simulink library "sm_wheel_loader_lib"  (R2026a)
settings: Solver=VariableStepAuto
undefined symbols (not defined in the file): AToTOrificeVector, BiPOrificeVector, boomHEArea, boomREArea, BToTOrificeVector, fluids, GRake, GToothL, GToothR, HMPST, HydFcnParams, logLoad, Position, PToAOrificeVector, PToBOrificeVector, RakeL, RakeR, testInput, Wheel_Loader, X, Y, Z
libraries: sm_lib x694, fl_lib x183, nesl_utility x74, SimscapeFluids_lib x62, sdl_lib x25, cvt_components_lib x25, simulink_extras x5, $bdroot x4, wheel_loader_contact_lib x4, ee_lib x2, SignalEditorBlockLib x1, batteryecm_lib x1
(part 5 of 25)

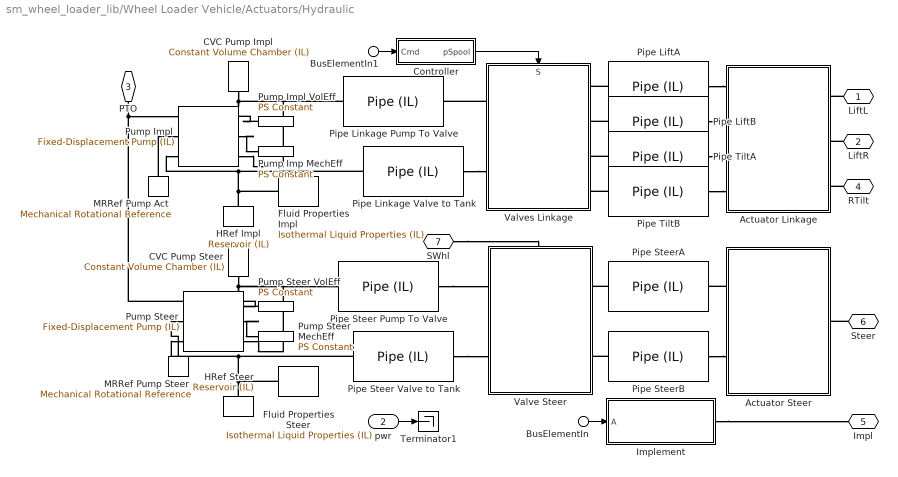
== system sm_wheel_loader_lib/Wheel Loader Vehicle/Actuators/Hydraulic ==
  BusElementIn : Inport  PortName=Cmd  Element=Actuator
  BusElementIn1 : Inport  PortName=Cmd  Element=Operator
  pwr : Inport  Port=2
  Actuator Linkage : Subsystem
      mask Display: image('sm_wheel_loader_actuator_linkage_IMAGE.png');
  Actuator Steer : Subsystem
      mask Display: image('sm_wheel_loader_actuator_steer_IMAGE.png');
  CVC Pump Impl : fl_lib/Isothermal Liquid/Elements/Constant Volume Chamber (IL)  volume=HydFcnParams.pump.chamberVol mm^3  p_I_specify=off  p_I_priority=High  p_I=0.101325 MPa  p_I_nominal_specify=off  p_I_nominal_value=1  p_I_nominal_unit=MPa
  CVC Pump Steer : fl_lib/Isothermal Liquid/Elements/Constant Volume Chamber (IL)  volume=HydFcnParams.steerPump.chamberVol mm^3  p_I_specify=off  p_I_priority=High  p_I=0.101325 MPa  p_I_nominal_specify=off  p_I_nominal_value=1  p_I_nominal_unit=MPa
  Controller : Subsystem
  Fluid Properties Impl : fl_lib/Isothermal Liquid/Utilities/Isothermal Liquid Properties (IL)  rho_L_atm=870 kg/m^3  bulk_modulus_model=foundation.enum.bulk_modulus_model.const  beta_gain=6  beta_L_atm=1.45e9 Pa  nu_atm=46 mm^2/s  p_atm=0.101325 MPa  p_min=0.1 Pa  properties_range_check=simscape.enum.assert.action.error  air_fraction=0.005  polytropic_index=1.0  rho_g_atm=1.225 kg/m^3  air_dissolution_model=simscape.enum.onoff.off  p_crit=3 MPa
  Fluid Properties Steer : fl_lib/Isothermal Liquid/Utilities/Isothermal Liquid Properties (IL)  rho_L_atm=870 kg/m^3  bulk_modulus_model=foundation.enum.bulk_modulus_model.const  beta_gain=6  beta_L_atm=1.45e9 Pa  nu_atm=46 mm^2/s  p_atm=0.101325 MPa  p_min=0.1 Pa  properties_range_check=simscape.enum.assert.action.error  air_fraction=0.005  polytropic_index=1.0  rho_g_atm=1.225 kg/m^3  air_dissolution_model=simscape.enum.onoff.off  p_crit=3 MPa
  HRef Impl : fl_lib/Isothermal Liquid/Elements/Reservoir (IL)  pressure_input=false  pressure_spec=foundation.enum.pressure_spec.atmospheric  reservoir_pressure=0.101325 MPa
  HRef Steer : fl_lib/Isothermal Liquid/Elements/Reservoir (IL)  pressure_input=false  pressure_spec=foundation.enum.pressure_spec.atmospheric  reservoir_pressure=0.101325 MPa
  Implement : Subsystem  Variant=on  VariantControlMode=label  VariantControl=Grapple Rake  LabelModeActiveChoice=Bucket
      settings: AttributesFormatString=%<LabelModeActiveChoice>
  MRRef Pump Act : fl_lib/Mechanical/Rotational Elements/Mechanical Rotational Reference
  MRRef Pump Steer : fl_lib/Mechanical/Rotational Elements/Mechanical Rotational Reference
  Pipe LiftA : fl_lib/Isothermal Liquid/Elements/Pipe (IL)  length=HydFcnParams.pipes.length mm  area=HydFcnParams.pipe.crossSectArea mm^2  Dh=HydFcnParams.pipes.hydraulicDiam mm  length_add=1 m  roughness=15e-6 m  Re_lam=2000  Re_tur=4000  shape_factor=64  dynamic_compressibility=simscape.enum.onoff.off  inertia=simscape.enum.onoff.off  p0=0.101325 MPa  mdot0=0 kg/s
  Pipe LiftB : fl_lib/Isothermal Liquid/Elements/Pipe (IL)  length=HydFcnParams.pipes.length mm  area=HydFcnParams.pipe.crossSectArea mm^2  Dh=HydFcnParams.pipes.hydraulicDiam mm  length_add=1 m  roughness=15e-6 m  Re_lam=2000  Re_tur=4000  shape_factor=64  dynamic_compressibility=simscape.enum.onoff.off  inertia=simscape.enum.onoff.off  p0=0.101325 MPa  mdot0=0 kg/s
  Pipe Linkage Pump To Valve : fl_lib/Isothermal Liquid/Elements/Pipe (IL)  length=HydFcnParams.pipes.length mm  area=HydFcnParams.pipe.crossSectArea mm^2  Dh=HydFcnParams.pipes.hydraulicDiam mm  length_add=1 m  roughness=15e-6 m  Re_lam=2000  Re_tur=4000  shape_factor=64  dynamic_compressibility=simscape.enum.onoff.off  inertia=simscape.enum.onoff.off  p0=0.101325 MPa  mdot0=0 kg/s
  Pipe Linkage Valve to Tank : fl_lib/Isothermal Liquid/Elements/Pipe (IL)  length=HydFcnParams.pipes.length mm  area=HydFcnParams.pipe.crossSectArea mm^2  Dh=HydFcnParams.pipes.hydraulicDiam mm  length_add=1 m  roughness=15e-6 m  Re_lam=2000  Re_tur=4000  shape_factor=64  dynamic_compressibility=simscape.enum.onoff.off  inertia=simscape.enum.onoff.off  p0=0.101325 MPa  mdot0=0 kg/s
  Pipe Steer Pump To Valve : fl_lib/Isothermal Liquid/Elements/Pipe (IL)  length=HydFcnParams.pipes.length mm  area=HydFcnParams.pipe.crossSectArea mm^2  Dh=HydFcnParams.pipes.hydraulicDiam mm  length_add=1 m  roughness=15e-6 m  Re_lam=2000  Re_tur=4000  shape_factor=64  dynamic_compressibility=simscape.enum.onoff.off  inertia=simscape.enum.onoff.off  p0=0.101325 MPa  mdot0=0 kg/s
  Pipe Steer Valve to Tank : fl_lib/Isothermal Liquid/Elements/Pipe (IL)  length=HydFcnParams.pipes.length mm  area=HydFcnParams.pipe.crossSectArea mm^2  Dh=HydFcnParams.pipes.hydraulicDiam mm  length_add=1 m  roughness=15e-6 m  Re_lam=2000  Re_tur=4000  shape_factor=64  dynamic_compressibility=simscape.enum.onoff.off  inertia=simscape.enum.onoff.off  p0=0.101325 MPa  mdot0=0 kg/s
  Pipe SteerA : fl_lib/Isothermal Liquid/Elements/Pipe (IL)  length=HydFcnParams.pipes.length mm  area=HydFcnParams.pipe.crossSectArea mm^2  Dh=HydFcnParams.pipes.hydraulicDiam mm  length_add=1 m  roughness=15e-6 m  Re_lam=2000  Re_tur=4000  shape_factor=64  dynamic_compressibility=simscape.enum.onoff.off  inertia=simscape.enum.onoff.off  p0=0.101325 MPa  mdot0=0 kg/s
  Pipe SteerB : fl_lib/Isothermal Liquid/Elements/Pipe (IL)  length=HydFcnParams.pipes.length mm  area=HydFcnParams.pipe.crossSectArea mm^2  Dh=HydFcnParams.pipes.hydraulicDiam mm  length_add=1 m  roughness=15e-6 m  Re_lam=2000  Re_tur=4000  shape_factor=64  dynamic_compressibility=simscape.enum.onoff.off  inertia=simscape.enum.onoff.off  p0=0.101325 MPa  mdot0=0 kg/s
  Pipe TiltA : fl_lib/Isothermal Liquid/Elements/Pipe (IL)  length=HydFcnParams.pipes.length mm  area=HydFcnParams.pipe.crossSectArea mm^2  Dh=HydFcnParams.pipes.hydraulicDiam mm  length_add=1 m  roughness=15e-6 m  Re_lam=2000  Re_tur=4000  shape_factor=64  dynamic_compressibility=simscape.enum.onoff.off  inertia=simscape.enum.onoff.off  p0=0.101325 MPa  mdot0=0 kg/s
  Pipe TiltB : fl_lib/Isothermal Liquid/Elements/Pipe (IL)  length=HydFcnParams.pipes.length mm  area=HydFcnParams.pipe.crossSectArea mm^2  Dh=HydFcnParams.pipes.hydraulicDiam mm  length_add=1 m  roughness=15e-6 m  Re_lam=2000  Re_tur=4000  shape_factor=64  dynamic_compressibility=simscape.enum.onoff.off  inertia=simscape.enum.onoff.off  p0=0.101325 MPa  mdot0=0 kg/s
  Pump Impl : SimscapeFluids_lib/Isothermal Liquid/Pumps & Motors/Fixed-Displacement Pump (IL)  leakage_friction_spec=fluids.isothermal_liquid.pumps_motors.enum.pump_motor_loss_spec.input_efficiency  displacement=HydFcnParams.pump.displacement cm^3/rev  omega_nominal=HydFcnParams.pump.nomSpeed rpm  p_nominal=HydFcnParams.pump.nomPrGain bar  vol_eff_nominal=HydFcnParams.pump.volEff  mech_eff_nominal=HydFcnParams.pump.mechEff  no_load_torque=0 N*m  p_diff_eff_TLU=[.1, 1, 2] MPa  omega_eff_TLU=[250, 500, 1000, 2000, 3000, 4000] rpm  vol_eff_TLU=[.816, .908, .954, .977, .981, .984; .325, .663, .831, .916, .925, .946; .137, .568, .78, .892, .893, .91]  mech_eff_TLU=[.996, .996, .996, .996, .996, .996; .988, .989, .989, .989, .989, .99; .981, .981, .982, .982, .983, .984]  p_diff_loss_TLU=[.1, 1, 2] MPa  omega_loss_TLU=[250, 500, 1000, 2000, 3000, 4000] rpm  vol_loss_TLU=1e-3 * [.023, .023, .023, .023, .0285, .032; .0844, .0842, .0845, .084, .1125, .108; .1079, .108, .11, .108, .1605, .18] m^3/s  mech_loss_TLU=[.002, .002, .002, .002, .002, .002; .0607, .0556, .0556, .0556, .0556, .0505; .1937, .1937, .1833, .1833, .1729, .1626] N*m  vol_eff_min=1e-3  vol_eff_max=1  mech_eff_min=1e-3  mech_eff_max=1  pressure_threshold=1e-3 MPa  omega_threshold=100 rpm  supplied_range_check=simscape.enum.assert.action.none  pump_mode_check=simscape.enum.assert.action.none  pressure_check=simscape.enum.assert.action.none  p_min_valid=0.101325 MPa
  Pump Steer : SimscapeFluids_lib/Isothermal Liquid/Pumps & Motors/Fixed-Displacement Pump (IL)  leakage_friction_spec=fluids.isothermal_liquid.pumps_motors.enum.pump_motor_loss_spec.input_efficiency  displacement=HydFcnParams.steerPump.displacement cm^3/rev  omega_nominal=HydFcnParams.pump.nomSpeed rpm  p_nominal=HydFcnParams.pump.nomPrGain bar  vol_eff_nominal=HydFcnParams.pump.volEff  mech_eff_nominal=HydFcnParams.pump.mechEff  no_load_torque=0 N*m  p_diff_eff_TLU=[.1, 1, 2] MPa  omega_eff_TLU=[250, 500, 1000, 2000, 3000, 4000] rpm  vol_eff_TLU=[.816, .908, .954, .977, .981, .984; .325, .663, .831, .916, .925, .946; .137, .568, .78, .892, .893, .91]  mech_eff_TLU=[.996, .996, .996, .996, .996, .996; .988, .989, .989, .989, .989, .99; .981, .981, .982, .982, .983, .984]  p_diff_loss_TLU=[.1, 1, 2] MPa  omega_loss_TLU=[250, 500, 1000, 2000, 3000, 4000] rpm  vol_loss_TLU=1e-3 * [.023, .023, .023, .023, .0285, .032; .0844, .0842, .0845, .084, .1125, .108; .1079, .108, .11, .108, .1605, .18] m^3/s  mech_loss_TLU=[.002, .002, .002, .002, .002, .002; .0607, .0556, .0556, .0556, .0556, .0505; .1937, .1937, .1833, .1833, .1729, .1626] N*m  vol_eff_min=1e-3  vol_eff_max=1  mech_eff_min=1e-3  mech_eff_max=1  pressure_threshold=1e-3 MPa  omega_threshold=100 rpm  supplied_range_check=simscape.enum.assert.action.none  pump_mode_check=simscape.enum.assert.action.none  pressure_check=simscape.enum.assert.action.none  p_min_valid=0.101325 MPa
  Pump Imp MechEff : fl_lib/Physical Signals/Sources/PS Constant  constant=HydFcnParams.pump.mechEff
  Pump Impl VolEff : fl_lib/Physical Signals/Sources/PS Constant  constant=HydFcnParams.pump.volEff
  Pump Steer MechEff : fl_lib/Physical Signals/Sources/PS Constant  constant=HydFcnParams.steerPump.mechEff
  Pump Steer VolEff : fl_lib/Physical Signals/Sources/PS Constant  constant=HydFcnParams.steerPump.volEff
  Terminator1 : Terminator
  Valve Steer : Subsystem
      settings: PortSchema="{\"entries\":[{\"content\":{\"sides\":[{\"content\":{\"connectorIds\":[\"LConn1\",\"LConn2\"]},\"type\":\"ConnectorPlacement.EquallySpacedRectSide\",\"uuid\":\"408e1035-6b3d-4519-b3f1-e009707ee901\"},{\"content\":{\"connectorIds\":[\"RConn1\",\"RConn2\"],\"side\":\"RIGHT\"},\"type\":\"ConnectorPlacement.EquallySpacedRectSide\",\"uuid\":\"f6fc5ec3-963d-4896-a810-4c1d83a284ca\"},{\"content\":{\"connectorIds\":[\"LConn3\"],\"side\":\"TOP\"},\"type\":\"ConnectorPlacement.EquallySpacedRectSide\",\"uuid\":\"5ee59ebc-e402-4785-9120-6ae47dd60b43\"},{\"content\":{\"side\":\"BOTTOM\"},\"type\":\"ConnectorPlacement.EquallySpacedRectSide\",\"uuid\":\"a994d606-c935-4c5d-b566-9fce03890d2a\"}]},\"type\":\"ConnectorPlacement.EquallySpacedConnector\",\"uuid\":\"c6791463-b308-429c-8dd1-d15f50199213\"}],\"packageUris\":[\"http://schema.mathworks.com/mf0/Connector/R2020b\"],\"version\":\"1.0\"}"
      mask Display: image('sm_wheel_loader_valve_gerotor_IMAGE.png');
  Valves Linkage : Subsystem
      settings: PortSchema="{\"entries\":[{\"content\":{\"sides\":[{\"content\":{\"connectorIds\":[\"LConn1\",\"LConn2\"]},\"type\":\"ConnectorPlacement.EquallySpacedRectSide\",\"uuid\":\"e97bc73b-9f55-4fad-8581-2066e0d00398\"},{\"content\":{\"connectorIds\":[\"RConn1\",\"RConn2\",\"RConn3\",\"RConn4\"],\"side\":\"RIGHT\"},\"type\":\"ConnectorPlacement.EquallySpacedRectSide\",\"uuid\":\"96a7ce6b-69e5-4ab0-8b6a-18f7c232fee9\"},{\"content\":{\"connectorIds\":[\"In1\"],\"side\":\"TOP\"},\"type\":\"ConnectorPlacement.EquallySpacedRectSide\",\"uuid\":\"ae84efc8-1053-4ca4-8a9f-7b6269b642b7\"}]},\"type\":\"ConnectorPlacement.EquallySpacedConnector\",\"uuid\":\"dc6a267f-cf26-460c-b9d1-1342509ba07b\"}],\"packageUris\":[\"http://schema.mathworks.com/mf0/Connector/R2020b\"],\"version\":\"1.0\"}"
      mask Display: image('sm_wheel_loader_valve_linkage_IMAGE.png');
  LiftL : PMIOPort  Side=Right
  LiftR : PMIOPort  Port=2  Side=Right
  PTO : PMIOPort  Port=3  Side=Left
  RTilt : PMIOPort  Port=4  Side=Left
  Impl : PMIOPort  Port=5  Side=Right
  Steer : PMIOPort  Port=6  Side=Right
  SWhl : PMIOPort  Port=7  Side=Left
  wires:
  BusElementIn1/1 -> Controller/1(Cmd)
  BusElementIn/1 -> Implement/1(A)
  Controller/1(pSpool) -> Valves Linkage/1(S)
  pwr/1 -> Terminator1/1
  connections:
  Pump Steer/RConn1 -- Pump Impl/RConn1 -- PTO/RConn1
  Implement/RConn1 -- Impl/RConn1
  Steer/RConn1 -- Actuator Steer/RConn1
  LiftR/RConn1 -- Actuator Linkage/RConn2
  MRRef Pump Steer/LConn1 -- Pump Steer/RConn2
  MRRef Pump Act/LConn1 -- Pump Impl/RConn2
  Pipe Steer Pump To Valve/RConn1 -- Valve Steer/LConn1
  Pump Steer/LConn2 -- Pump Steer MechEff/RConn1
  Pump Steer VolEff/RConn1 -- Pump Steer/LConn1
  Pipe Steer Valve to Tank/LConn1 -- Valve Steer/LConn2
  CVC Pump Steer/LConn1 -- Pump Steer/LConn3 -- Pipe Steer Pump To Valve/LConn1
  Fluid Properties Steer/RConn1 -- Pipe Steer Valve to Tank/RConn1 -- Pump Steer/RConn3 -- HRef Steer/LConn1
  Pipe SteerB/LConn1 -- Valve Steer/RConn2
  Pipe SteerA/LConn1 -- Valve Steer/RConn1
  RTilt/RConn1 -- Actuator Linkage/RConn3
  Actuator Steer/LConn1 -- Pipe SteerA/RConn1
  Pipe SteerB/RConn1 -- Actuator Steer/LConn2
  Pipe TiltB/RConn1 -- Actuator Linkage/LConn4
  Pipe TiltA/RConn1 -- Actuator Linkage/LConn3
  Pipe LiftB/RConn1 -- Actuator Linkage/LConn2
  Pipe LiftA/RConn1 -- Actuator Linkage/LConn1
  LiftL/RConn1 -- Actuator Linkage/RConn1
  Pipe TiltB/LConn1 -- Valves Linkage/RConn4
  Pipe TiltA/LConn1 -- Valves Linkage/RConn3
  Pipe LiftB/LConn1 -- Valves Linkage/RConn2
  Pipe LiftA/LConn1 -- Valves Linkage/RConn1
  Pipe Linkage Valve to Tank/LConn1 -- Valves Linkage/LConn2
  Valves Linkage/LConn1 -- Pipe Linkage Pump To Valve/RConn1
  HRef Impl/LConn1 -- Pipe Linkage Valve to Tank/RConn1 -- Pump Impl/RConn3 -- Fluid Properties Impl/RConn1
  Pipe Linkage Pump To Valve/LConn1 -- Pump Impl/LConn3 -- CVC Pump Impl/LConn1
  Pump Impl/LConn2 -- Pump Imp MechEff/RConn1
  Pump Impl VolEff/RConn1 -- Pump Impl/LConn1
  SWhl/RConn1 -- Valve Steer/LConn3

== system sm_wheel_loader_lib/Wheel Loader Vehicle/Actuators/Ideal ==
  note: The actuation of the cylinders is done through prescribed motion at the joints.
  Cmd : Inport
  pwr : Inport  Port=2
  Power Draw : Subsystem
  Shaft Inertia : fl_lib/Mechanical/Rotational Elements/Inertia  inertia=0.01 kg*m^2  num_ports=foundation.enum.numPorts2.one  w_specify=on  w_priority=None  w=0 rad/s  w_nominal_specify=off  w_nominal_value=1  w_nominal_unit=rad/s  t_specify=off  t_priority=None  t=0 N*m  t_nominal_specify=off  t_nominal_value=1  t_nominal_unit=N*m
  Steering Mechanism Inertia : fl_lib/Mechanical/Rotational Elements/Inertia  inertia=0.01 kg*m^2  num_ports=foundation.enum.numPorts2.one  w_specify=off  w_priority=High  w=0 rad/s  w_nominal_specify=off  w_nominal_value=1  w_nominal_unit=rad/s  t_specify=off  t_priority=None  t=0 N*m  t_nominal_specify=off  t_nominal_value=1  t_nominal_unit=N*m
  Terminator : Terminator
  LiftL : PMIOPort  Side=Right
  LiftR : PMIOPort  Port=2  Side=Right
  PTO : PMIOPort  Port=3  Side=Left
  RTilt : PMIOPort  Port=4  Side=Left
  Impl : PMIOPort  Port=5  Side=Right
  Steer : PMIOPort  Port=6  Side=Right
  SWhl : PMIOPort  Port=7  Side=Left
  wires:
  Cmd/1 -> Terminator/1
  pwr/1 -> Power Draw/1(pwr)
  connections:
  PTO/RConn1 -- Power Draw/RConn1 -- Shaft Inertia/LConn1
  Steering Mechanism Inertia/LConn1 -- SWhl/RConn1

== system sm_wheel_loader_lib/Wheel Loader Vehicle/Driveline/Axle Housing Front ==
  Bearing : sm_lib/Body Elements/File Solid  ExtGeomFileName=AxleF_Housing_Bearing.STEP  UnitType=FromFile  ExtGeomFileUnits=m  StepReaderType=HEX  ExportConvexHullGeometry=off  InertiaType=Custom  BasedOnType=DensityFromFile  Density=1000  DensityUnits=kg/m^3  Mass=Wheel_Loader.bodyGroups(36).subGroups(2).inertialProperties.mass  MassUnits=kg  CenterOfMass=Wheel_Loader.bodyGroups(36).subGroups(2).inertialProperties.centerOfMass  CenterOfMassUnits=m  MomentsOfInertia=Wheel_Loader.bodyGroups(36).subGroups(2).inertialProperties.momentsOfInertia  MomentsOfInertiaUnits=kg*m^2  ProductsOfInertia=Wheel_Loader.bodyGroups(36).subGroups(2).inertialProperties.productsOfInertia  ProductsOfInertiaUnits=kg*m^2  GraphicType=FromGeometry  MarkerShape=Sphere  MarkerSize=10  GraphicVisPropType=SimpleVisualProperties  GraphicDiffuseColor=Wheel_Loader.bodyGroups(36).subGroups(2).visualProperties.rgb  GraphicOpacity=fa_casing_opc  GraphicSpecularColor=[0.5 0.5 0.5 1.0]  GraphicAmbientColor=[0.15 0.15 0.15 1.0]  GraphicEmissiveColor=[0.0 0.0 0.0 1.0]  GraphicShininess=75  DoExposeReferenceFrame=on  SerializedFrames=<Frames/>
  Bolts : sm_lib/Body Elements/File Solid  ExtGeomFileName=AxleF_Housing_Bolts.STEP  UnitType=FromFile  ExtGeomFileUnits=m  StepReaderType=HEX  ExportConvexHullGeometry=off  InertiaType=Custom  BasedOnType=DensityFromFile  Density=1000  DensityUnits=kg/m^3  Mass=Wheel_Loader.bodyGroups(36).subGroups(3).inertialProperties.mass  MassUnits=kg  CenterOfMass=Wheel_Loader.bodyGroups(36).subGroups(3).inertialProperties.centerOfMass  CenterOfMassUnits=m  MomentsOfInertia=Wheel_Loader.bodyGroups(36).subGroups(3).inertialProperties.momentsOfInertia  MomentsOfInertiaUnits=kg*m^2  ProductsOfInertia=Wheel_Loader.bodyGroups(36).subGroups(3).inertialProperties.productsOfInertia  ProductsOfInertiaUnits=kg*m^2  GraphicType=FromGeometry  MarkerShape=Sphere  MarkerSize=10  GraphicVisPropType=SimpleVisualProperties  GraphicDiffuseColor=Wheel_Loader.bodyGroups(36).subGroups(3).visualProperties.rgb  GraphicOpacity=fa_casing_opc  GraphicSpecularColor=[0.5 0.5 0.5 1.0]  GraphicAmbientColor=[0.15 0.15 0.15 1.0]  GraphicEmissiveColor=[0.0 0.0 0.0 1.0]  GraphicShininess=75  DoExposeReferenceFrame=on  SerializedFrames=<Frames/>
  Housing : sm_lib/Body Elements/File Solid  ExtGeomFileName=AxleF_Housing.STEP  UnitType=FromFile  ExtGeomFileUnits=m  StepReaderType=HEX  ExportConvexHullGeometry=off  InertiaType=Custom  BasedOnType=DensityFromFile  Density=1000  DensityUnits=kg/m^3  Mass=Wheel_Loader.bodyGroups(36).subGroups(1).inertialProperties.mass  MassUnits=kg  CenterOfMass=Wheel_Loader.bodyGroups(36).subGroups(1).inertialProperties.centerOfMass  CenterOfMassUnits=m  MomentsOfInertia=Wheel_Loader.bodyGroups(36).subGroups(1).inertialProperties.momentsOfInertia  MomentsOfInertiaUnits=kg*m^2  ProductsOfInertia=Wheel_Loader.bodyGroups(36).subGroups(1).inertialProperties.productsOfInertia  ProductsOfInertiaUnits=kg*m^2  GraphicType=FromGeometry  MarkerShape=Sphere  MarkerSize=10  GraphicVisPropType=SimpleVisualProperties  GraphicDiffuseColor=Wheel_Loader.bodyGroups(36).subGroups(1).visualProperties.rgb  GraphicOpacity=fa_casing_opc  GraphicSpecularColor=[0.5 0.5 0.5 1.0]  GraphicAmbientColor=[0.15 0.15 0.15 1.0]  GraphicEmissiveColor=[0.0 0.0 0.0 1.0]  GraphicShininess=75  DoExposeReferenceFrame=on  SerializedFrames=<Frames/>
  RT_FrontAxle_FDPinion : sm_lib/Frames and Transforms/Rigid Transform  RotationMethod=RotationMatrix  FollAlignAxisA=+X  BaseAlignAxisA=+Y  FollAlignAxisB=+Y  BaseAlignAxisB=+Z  RotationStandardAxis=+Z  RotationAngle=0.0  RotationAngleUnits=deg  RotationArbitraryAxis=[0 0 1]  RotationSequenceAxes=FollowerAxes  RotationSequence=XYX  RotationSequenceAngles=[0 0 0]  RotationSequenceAnglesUnits=deg  RotationMatrix=Wheel_Loader.coordSys(44).transform.rotation  Quaternion=[1 0 0 0]  TranslationMethod=Cartesian  TranslationCartesianOffset=Wheel_Loader.coordSys(44).transform.translation  TranslationCartesianOffsetUnits=m  TranslationStandardAxis=+Z  TranslationStandardOffset=0  TranslationStandardOffsetUnits=m  TranslationROffset=0  TranslationROffsetUnits=m  TranslationThetaOffset=0  TranslationThetaOffsetUnits=deg  TranslationZOffset=0  TranslationZOffsetUnits=m
  RT_FrontAxle_LFFDRing_Weld : sm_lib/Frames and Transforms/Rigid Transform  RotationMethod=RotationMatrix  FollAlignAxisA=+X  BaseAlignAxisA=+Y  FollAlignAxisB=+Y  BaseAlignAxisB=+Z  RotationStandardAxis=+Z  RotationAngle=0.0  RotationAngleUnits=deg  RotationArbitraryAxis=[0 0 1]  RotationSequenceAxes=FollowerAxes  RotationSequence=XYX  RotationSequenceAngles=[0 0 0]  RotationSequenceAnglesUnits=deg  RotationMatrix=Wheel_Loader.coordSys(70).transform.rotation  Quaternion=[1 0 0 0]  TranslationMethod=Cartesian  TranslationCartesianOffset=Wheel_Loader.coordSys(70).transform.translation  TranslationCartesianOffsetUnits=m  TranslationStandardAxis=+Z  TranslationStandardOffset=0  TranslationStandardOffsetUnits=m  TranslationROffset=0  TranslationROffsetUnits=m  TranslationThetaOffset=0  TranslationThetaOffsetUnits=deg  TranslationZOffset=0  TranslationZOffsetUnits=m
  RT_FrontAxle_RFFDRing_Weld : sm_lib/Frames and Transforms/Rigid Transform  RotationMethod=RotationMatrix  FollAlignAxisA=+X  BaseAlignAxisA=+Y  FollAlignAxisB=+Y  BaseAlignAxisB=+Z  RotationStandardAxis=+Z  RotationAngle=0.0  RotationAngleUnits=deg  RotationArbitraryAxis=[0 0 1]  RotationSequenceAxes=FollowerAxes  RotationSequence=XYX  RotationSequenceAngles=[0 0 0]  RotationSequenceAnglesUnits=deg  RotationMatrix=Wheel_Loader.coordSys(66).transform.rotation  Quaternion=[1 0 0 0]  TranslationMethod=Cartesian  TranslationCartesianOffset=Wheel_Loader.coordSys(66).transform.translation  TranslationCartesianOffsetUnits=m  TranslationStandardAxis=+Z  TranslationStandardOffset=0  TranslationStandardOffsetUnits=m  TranslationROffset=0  TranslationROffsetUnits=m  TranslationThetaOffset=0  TranslationThetaOffsetUnits=deg  TranslationZOffset=0  TranslationZOffsetUnits=m
  RT_FrontFrame_Axle_Weld : sm_lib/Frames and Transforms/Rigid Transform  RotationMethod=RotationMatrix  FollAlignAxisA=+X  BaseAlignAxisA=+Y  FollAlignAxisB=+Y  BaseAlignAxisB=+Z  RotationStandardAxis=+Z  RotationAngle=0.0  RotationAngleUnits=deg  RotationArbitraryAxis=[0 0 1]  RotationSequenceAxes=FollowerAxes  RotationSequence=XYX  RotationSequenceAngles=[0 0 0]  RotationSequenceAnglesUnits=deg  RotationMatrix=[1 0 0; 0 1 0; 0 0 1]  Quaternion=[1 0 0 0]  TranslationMethod=Cartesian  TranslationCartesianOffset=[0 0 0]  TranslationCartesianOffsetUnits=m  TranslationStandardAxis=+Z  TranslationStandardOffset=0  TranslationStandardOffsetUnits=m  TranslationROffset=0  TranslationROffsetUnits=m  TranslationThetaOffset=0  TranslationThetaOffsetUnits=deg  TranslationZOffset=0  TranslationZOffsetUnits=m
  HFL : PMIOPort  Side=Left
  Frame : PMIOPort  Port=2  Side=Right
  HFP : PMIOPort  Port=3  Side=Left
  HFR : PMIOPort  Port=4  Side=Left
  connections:
  RT_FrontAxle_LFFDRing_Weld/RConn1 -- HFL/RConn1
  RT_FrontAxle_RFFDRing_Weld/RConn1 -- HFR/RConn1
  RT_FrontAxle_FDPinion/RConn1 -- HFP/RConn1
  RT_FrontFrame_Axle_Weld/RConn1 -- Frame/RConn1
  Housing/RConn1 -- Bolts/RConn1 -- Bearing/RConn1 -- RT_FrontFrame_Axle_Weld/LConn1 -- RT_FrontAxle_FDPinion/LConn1 -- RT_FrontAxle_RFFDRing_Weld/LConn1 -- RT_FrontAxle_LFFDRing_Weld/LConn1

== system sm_wheel_loader_lib/Wheel Loader Vehicle/Driveline/Axle Housing Rear ==
  Bolts : sm_lib/Body Elements/File Solid  ExtGeomFileName=AxleR_Housing_Bolts.STEP  UnitType=FromFile  ExtGeomFileUnits=m  StepReaderType=HEX  ExportConvexHullGeometry=off  InertiaType=Custom  BasedOnType=DensityFromFile  Density=1000  DensityUnits=kg/m^3  Mass=Wheel_Loader.bodyGroups(37).subGroups(2).inertialProperties.mass  MassUnits=kg  CenterOfMass=Wheel_Loader.bodyGroups(37).subGroups(2).inertialProperties.centerOfMass  CenterOfMassUnits=m  MomentsOfInertia=Wheel_Loader.bodyGroups(37).subGroups(2).inertialProperties.momentsOfInertia  MomentsOfInertiaUnits=kg*m^2  ProductsOfInertia=Wheel_Loader.bodyGroups(37).subGroups(2).inertialProperties.productsOfInertia  ProductsOfInertiaUnits=kg*m^2  GraphicType=FromGeometry  MarkerShape=Sphere  MarkerSize=10  GraphicVisPropType=SimpleVisualProperties  GraphicDiffuseColor=Wheel_Loader.bodyGroups(37).subGroups(2).visualProperties.rgb  GraphicOpacity=ra_casing_opc  GraphicSpecularColor=[0.5 0.5 0.5 1.0]  GraphicAmbientColor=[0.15 0.15 0.15 1.0]  GraphicEmissiveColor=[0.0 0.0 0.0 1.0]  GraphicShininess=75  DoExposeReferenceFrame=on  SerializedFrames=<Frames/>
  Housing : sm_lib/Body Elements/File Solid  ExtGeomFileName=AxleR_Housing.STEP  UnitType=FromFile  ExtGeomFileUnits=m  StepReaderType=HEX  ExportConvexHullGeometry=off  InertiaType=Custom  BasedOnType=DensityFromFile  Density=1000  DensityUnits=kg/m^3  Mass=Wheel_Loader.bodyGroups(37).subGroups(1).inertialProperties.mass  MassUnits=kg  CenterOfMass=Wheel_Loader.bodyGroups(37).subGroups(1).inertialProperties.centerOfMass  CenterOfMassUnits=m  MomentsOfInertia=Wheel_Loader.bodyGroups(37).subGroups(1).inertialProperties.momentsOfInertia  MomentsOfInertiaUnits=kg*m^2  ProductsOfInertia=Wheel_Loader.bodyGroups(37).subGroups(1).inertialProperties.productsOfInertia  ProductsOfInertiaUnits=kg*m^2  GraphicType=FromGeometry  MarkerShape=Sphere  MarkerSize=10  GraphicVisPropType=SimpleVisualProperties  GraphicDiffuseColor=Wheel_Loader.bodyGroups(37).subGroups(1).visualProperties.rgb  GraphicOpacity=ra_casing_opc  GraphicSpecularColor=[0.5 0.5 0.5 1.0]  GraphicAmbientColor=[0.15 0.15 0.15 1.0]  GraphicEmissiveColor=[0.0 0.0 0.0 1.0]  GraphicShininess=75  DoExposeReferenceFrame=on  SerializedFrames=<Frames/>
  RT_RearAxle_GBHousing_Weld : sm_lib/Frames and Transforms/Rigid Transform  RotationMethod=RotationMatrix  FollAlignAxisA=+X  BaseAlignAxisA=+Y  FollAlignAxisB=+Y  BaseAlignAxisB=+Z  RotationStandardAxis=+Z  RotationAngle=0.0  RotationAngleUnits=deg  RotationArbitraryAxis=[0 0 1]  RotationSequenceAxes=FollowerAxes  RotationSequence=XYX  RotationSequenceAngles=[0 0 0]  RotationSequenceAnglesUnits=deg  RotationMatrix=Wheel_Loader.coordSys(56).transform.rotation  Quaternion=[1 0 0 0]  TranslationMethod=Cartesian  TranslationCartesianOffset=Wheel_Loader.coordSys(56).transform.translation  TranslationCartesianOffsetUnits=m  TranslationStandardAxis=+Z  TranslationStandardOffset=0  TranslationStandardOffsetUnits=m  TranslationROffset=0  TranslationROffsetUnits=m  TranslationThetaOffset=0  TranslationThetaOffsetUnits=deg  TranslationZOffset=0  TranslationZOffsetUnits=m
  RT_RearAxle_LRFDRing_Weld : sm_lib/Frames and Transforms/Rigid Transform  RotationMethod=RotationMatrix  FollAlignAxisA=+X  BaseAlignAxisA=+Y  FollAlignAxisB=+Y  BaseAlignAxisB=+Z  RotationStandardAxis=+Z  RotationAngle=0.0  RotationAngleUnits=deg  RotationArbitraryAxis=[0 0 1]  RotationSequenceAxes=FollowerAxes  RotationSequence=XYX  RotationSequenceAngles=[0 0 0]  RotationSequenceAnglesUnits=deg  RotationMatrix=Wheel_Loader.coordSys(62).transform.rotation  Quaternion=[1 0 0 0]  TranslationMethod=Cartesian  TranslationCartesianOffset=Wheel_Loader.coordSys(62).transform.translation  TranslationCartesianOffsetUnits=m  TranslationStandardAxis=+Z  TranslationStandardOffset=0  TranslationStandardOffsetUnits=m  TranslationROffset=0  TranslationROffsetUnits=m  TranslationThetaOffset=0  TranslationThetaOffsetUnits=deg  TranslationZOffset=0  TranslationZOffsetUnits=m
  RT_RearAxle_RRFDRing_Weld : sm_lib/Frames and Transforms/Rigid Transform  RotationMethod=RotationMatrix  FollAlignAxisA=+X  BaseAlignAxisA=+Y  FollAlignAxisB=+Y  BaseAlignAxisB=+Z  RotationStandardAxis=+Z  RotationAngle=0.0  RotationAngleUnits=deg  RotationArbitraryAxis=[0 0 1]  RotationSequenceAxes=FollowerAxes  RotationSequence=XYX  RotationSequenceAngles=[0 0 0]  RotationSequenceAnglesUnits=deg  RotationMatrix=Wheel_Loader.coordSys(58).transform.rotation  Quaternion=[1 0 0 0]  TranslationMethod=Cartesian  TranslationCartesianOffset=Wheel_Loader.coordSys(58).transform.translation  TranslationCartesianOffsetUnits=m  TranslationStandardAxis=+Z  TranslationStandardOffset=0  TranslationStandardOffsetUnits=m  TranslationROffset=0  TranslationROffsetUnits=m  TranslationThetaOffset=0  TranslationThetaOffsetUnits=deg  TranslationZOffset=0  TranslationZOffsetUnits=m
  RT_RearFrame_Axle_Weld : sm_lib/Frames and Transforms/Rigid Transform  RotationMethod=RotationMatrix  FollAlignAxisA=+X  BaseAlignAxisA=+Y  FollAlignAxisB=+Y  BaseAlignAxisB=+Z  RotationStandardAxis=+Z  RotationAngle=0.0  RotationAngleUnits=deg  RotationArbitraryAxis=[0 0 1]  RotationSequenceAxes=FollowerAxes  RotationSequence=XYX  RotationSequenceAngles=[0 0 0]  RotationSequenceAnglesUnits=deg  RotationMatrix=[1 0 0; 0 1 0; 0 0 1]  Quaternion=[1 0 0 0]  TranslationMethod=Cartesian  TranslationCartesianOffset=[0 0 0]  TranslationCartesianOffsetUnits=m  TranslationStandardAxis=+Z  TranslationStandardOffset=0  TranslationStandardOffsetUnits=m  TranslationROffset=0  TranslationROffsetUnits=m  TranslationThetaOffset=0  TranslationThetaOffsetUnits=deg  TranslationZOffset=0  TranslationZOffsetUnits=m
  Frame : PMIOPort  Side=Left
  HRL : PMIOPort  Port=2  Side=Right
  HRP : PMIOPort  Port=3  Side=Right
  HRR : PMIOPort  Port=4  Side=Right
  connections:
  RT_RearAxle_LRFDRing_Weld/RConn1 -- HRL/RConn1
  RT_RearAxle_RRFDRing_Weld/RConn1 -- HRR/RConn1
  RT_RearAxle_GBHousing_Weld/RConn1 -- HRP/RConn1
  RT_RearFrame_Axle_Weld/RConn1 -- Frame/RConn1
  RT_RearAxle_RRFDRing_Weld/LConn1 -- RT_RearAxle_LRFDRing_Weld/LConn1 -- Housing/RConn1 -- Bolts/RConn1 -- RT_RearFrame_Axle_Weld/LConn1 -- RT_RearAxle_GBHousing_Weld/LConn1

== system sm_wheel_loader_lib/Wheel Loader Vehicle/Driveline/Driveline ==
  Driveline 1D : Subsystem  VariantControl=Driveline_1D
      settings: PortSchema="{\"entries\":[{\"content\":{\"sides\":[{\"content\":{\"connectorIds\":[\"LConn1\",\"LConn2\",\"LConn3\"]},\"type\":\"ConnectorPlacement.EquallySpacedRectSide\",\"uuid\":\"b63b559c-62bd-445e-b7ec-d91a1cc2405e\"},{\"content\":{\"connectorIds\":[\"RConn1\",\"RConn2\",\"RConn3\"],\"side\":\"RIGHT\"},\"type\":\"ConnectorPlacement.EquallySpacedRectSide\",\"uuid\":\"032d5054-ea2a-4303-8f34-205eab6388de\"},{\"content\":{\"connectorIds\":[\"LConn4\",\"LConn5\",\"LConn6\"],\"side\":\"TOP\"},\"type\":\"ConnectorPlacement.EquallySpacedRectSide\",\"uuid\":\"d2f0756e-9d37-498a-a5f3-0e74497a6223\"},{\"content\":{\"connectorIds\":[\"RConn4\",\"RConn5\",\"RConn6\"],\"side\":\"BOTTOM\"},\"type\":\"ConnectorPlacement.EquallySpacedRectSide\",\"uuid\":\"6a60c5c4-76fc-4699-b9fc-b8ae6c8913a6\"}]},\"type\":\"ConnectorPlacement.EquallySpacedConnector\",\"uuid\":\"1dc94a05-d7e7-41ec-b5c7-4a84600f46a8\"}],\"packageUris\":[\"http://schema.mathworks.com/mf0/Connector/R2020b\"],\"version\":\"1.0\"}"
      mask Display: image('sm_wheel_loader_driveline1D_IMAGE.png')
  Driveline 3D : Subsystem  VariantControl=Driveline_3D  mask{popup_driveJointF=CV Joint, popup_driveJointR=CV Joint}
      mask prompts: popup_driveJointF "Driveshaft Joint (front)"; popup_driveJointR "Driveshaft Joint (rear)"
      settings: PortSchema="{\"entries\":[{\"content\":{\"sides\":[{\"content\":{\"connectorIds\":[\"LConn1\",\"LConn2\",\"LConn3\"]},\"type\":\"ConnectorPlacement.EquallySpacedRectSide\",\"uuid\":\"ac94f403-7500-4d3b-9e0f-075c8f20a849\"},{\"content\":{\"connectorIds\":[\"RConn1\",\"RConn2\",\"RConn3\"],\"side\":\"RIGHT\"},\"type\":\"ConnectorPlacement.EquallySpacedRectSide\",\"uuid\":\"0eb844aa-00af-4edc-a570-50ab4e6b66c2\"},{\"content\":{\"connectorIds\":[\"LConn4\",\"LConn5\",\"LConn6\"],\"side\":\"TOP\"},\"type\":\"ConnectorPlacement.EquallySpacedRectSide\",\"uuid\":\"abddfcb0-9899-4667-9404-ac15e4716921\"},{\"content\":{\"connectorIds\":[\"RConn4\",\"RConn5\",\"RConn6\"],\"side\":\"BOTTOM\"},\"type\":\"ConnectorPlacement.EquallySpacedRectSide\",\"uuid\":\"a33fa760-6818-409d-ace3-b40bc7e3acff\"}]},\"type\":\"ConnectorPlacement.EquallySpacedConnector\",\"uuid\":\"2bc03850-1261-46ce-b9b6-2dbda85e9fb0\"}],\"packageUris\":[\"http://schema.mathworks.com/mf0/Connector/R2020b\"],\"version\":\"1.0\"}"
      mask TypeOptions popup_driveJointF:
      | Driveshaft
      | Front/popup_driveJointF
      mask TypeOptions popup_driveJointR:
      | Driveshaft
      | Rear/popup_driveJointR
      mask Display: image('sm_wheel_loader_driveline3D_IMAGE.png')
  wRL : PMIOPort  Side=Left
  Tr1 : PMIOPort  Port=2  Side=Left
  wFL : PMIOPort  Port=3  Side=Left
  HRL : PMIOPort  Port=4  Side=Left
  HRP : PMIOPort  Port=5  Side=Left
  HRR : PMIOPort  Port=6  Side=Left
  wRR : PMIOPort  Port=7  Side=Right
  Tr : PMIOPort  Port=8  Side=Right
  wFR : PMIOPort  Port=9  Side=Right
  HFL : PMIOPort  Port=10  Side=Right
  HFP : PMIOPort  Port=11  Side=Right
  HFR : PMIOPort  Port=12  Side=Right

== system sm_wheel_loader_lib/Wheel Loader Vehicle/Driveline/Wheel FL ==
  Hub : Subsystem  Tag=B230D770-3EF4-C446-A53F-6306E8DE466B
  Tire : Subsystem  Tag=1B5B75A7-7B5C-4849-8411-0061864F750D
  C : PMIOPort  Side=Left
  S : PMIOPort  Port=2  Side=Right
  connections:
  S/RConn1 -- Hub/LConn1
  Tire/LConn1 -- Hub/RConn1
  C/RConn1 -- Tire/RConn1

== system sm_wheel_loader_lib/Wheel Loader Vehicle/Driveline/Wheel FR ==
  Hub : Subsystem  Tag=5DF5B1C3-69E9-F644-9747-64BA6A51FD34
  Tire : Subsystem  Tag=2A7E39F9-3B28-3A4E-B0C7-8D7EA453C230
  S : PMIOPort  Side=Left
  C : PMIOPort  Port=2  Side=Right
  connections:
  S/RConn1 -- Hub/LConn1
  C/RConn1 -- Tire/RConn1
  Tire/LConn1 -- Hub/RConn1

== system sm_wheel_loader_lib/Wheel Loader Vehicle/Driveline/Wheel RL ==
  Hub : Subsystem  Tag=CC0284A2-2BFF-0E47-890D-925832CDD082
  Tire : Subsystem  Tag=72D24446-88E9-5644-B0BB-80BAAAD3866B
  C : PMIOPort  Side=Left
  S : PMIOPort  Port=2  Side=Right
  connections:
  C/RConn1 -- Tire/RConn1
  Tire/LConn1 -- Hub/RConn1
  S/RConn1 -- Hub/LConn1

== system sm_wheel_loader_lib/Wheel Loader Vehicle/Driveline/Wheel RR ==
  Hub : Subsystem  Tag=11A7BD13-C7ED-8E4B-96CC-E8FBD77457E9
  Tire : Subsystem  Tag=1C442381-0767-DA43-BB70-3697AC20F422
  S : PMIOPort  Side=Left
  C : PMIOPort  Port=2  Side=Right
  connections:
  S/RConn1 -- Hub/LConn1
  C/RConn1 -- Tire/RConn1
  Hub/RConn1 -- Tire/LConn1

== system sm_wheel_loader_lib/Wheel Loader Vehicle/Frame Front/Camera Frames ==
  Reference Camera Cab : sm_lib/Frames and Transforms/Reference Frame
  Reference Camera ImplRR : sm_lib/Frames and Transforms/Reference Frame
  Reference Camera IsoFR : sm_lib/Frames and Transforms/Reference Frame
  Reference Camera LinkageR : sm_lib/Frames and Transforms/Reference Frame
  Reference Camera RR : sm_lib/Frames and Transforms/Reference Frame
  Reference Camera Rear : sm_lib/Frames and Transforms/Reference Frame
  Reference Camera Right : sm_lib/Frames and Transforms/Reference Frame
  Reference Camera Roof : sm_lib/Frames and Transforms/Reference Frame
  Reference Camera WhlFR : sm_lib/Frames and Transforms/Reference Frame
  Transform Camera Cab : sm_lib/Frames and Transforms/Rigid Transform  RotationMethod=None  FollAlignAxisA=+X  BaseAlignAxisA=+Y  FollAlignAxisB=+Y  BaseAlignAxisB=+Z  RotationStandardAxis=+Z  RotationAngle=0.0  RotationAngleUnits=deg  RotationArbitraryAxis=[0 0 1]  RotationSequenceAxes=FollowerAxes  RotationSequence=XYX  RotationSequenceAngles=[0 0 0]  RotationSequenceAnglesUnits=deg  RotationMatrix=[1 0 0; 0 1 0; 0 0 1]  Quaternion=[1 0 0 0]  TranslationMethod=Cartesian  TranslationCartesianOffset=[0 -0.75 1]  TranslationCartesianOffsetUnits=m  TranslationStandardAxis=+Z  TranslationStandardOffset=0  TranslationStandardOffsetUnits=m  TranslationROffset=0  TranslationROffsetUnits=m  TranslationThetaOffset=0  TranslationThetaOffsetUnits=deg  TranslationZOffset=0  TranslationZOffsetUnits=m
  Transform Camera ImplRR : sm_lib/Frames and Transforms/Rigid Transform  RotationMethod=StandardAxis  FollAlignAxisA=+X  BaseAlignAxisA=+Y  FollAlignAxisB=+Y  BaseAlignAxisB=+Z  RotationStandardAxis=+Z  RotationAngle=+15+90  RotationAngleUnits=deg  RotationArbitraryAxis=[0 0 1]  RotationSequenceAxes=FollowerAxes  RotationSequence=XYX  RotationSequenceAngles=[0 0 0]  RotationSequenceAnglesUnits=deg  RotationMatrix=[1 0 0; 0 1 0; 0 0 1]  Quaternion=[1 0 0 0]  TranslationMethod=Cartesian  TranslationCartesianOffset=[1.0 -0.5 0.75]  TranslationCartesianOffsetUnits=m  TranslationStandardAxis=+Z  TranslationStandardOffset=0  TranslationStandardOffsetUnits=m  TranslationROffset=0  TranslationROffsetUnits=m  TranslationThetaOffset=0  TranslationThetaOffsetUnits=deg  TranslationZOffset=0  TranslationZOffsetUnits=m
  Transform Camera IsoFR : sm_lib/Frames and Transforms/Rigid Transform  RotationMethod=RotationSequence  FollAlignAxisA=+X  BaseAlignAxisA=+Y  FollAlignAxisB=+Y  BaseAlignAxisB=+Z  RotationStandardAxis=+Z  RotationAngle=0.0  RotationAngleUnits=deg  RotationArbitraryAxis=[0 0 1]  RotationSequenceAxes=FollowerAxes  RotationSequence=ZYX  RotationSequenceAngles=[45 -20 0]  RotationSequenceAnglesUnits=deg  RotationMatrix=[1 0 0; 0 1 0; 0 0 1]  Quaternion=[1 0 0 0]  TranslationMethod=Cartesian  TranslationCartesianOffset=[3.2 4.0 2]  TranslationCartesianOffsetUnits=m  TranslationStandardAxis=+Z  TranslationStandardOffset=0  TranslationStandardOffsetUnits=m  TranslationROffset=0  TranslationROffsetUnits=m  TranslationThetaOffset=0  TranslationThetaOffsetUnits=deg  TranslationZOffset=0  TranslationZOffsetUnits=m
  Transform Camera LinkageR : sm_lib/Frames and Transforms/Rigid Transform  RotationMethod=None  FollAlignAxisA=+X  BaseAlignAxisA=+Y  FollAlignAxisB=+Y  BaseAlignAxisB=+Z  RotationStandardAxis=+Z  RotationAngle=0.0  RotationAngleUnits=deg  RotationArbitraryAxis=[0 0 1]  RotationSequenceAxes=FollowerAxes  RotationSequence=XYX  RotationSequenceAngles=[0 0 0]  RotationSequenceAnglesUnits=deg  RotationMatrix=[1 0 0; 0 1 0; 0 0 1]  Quaternion=[1 0 0 0]  TranslationMethod=Cartesian  TranslationCartesianOffset=[1.4 0.7 1]  TranslationCartesianOffsetUnits=m  TranslationStandardAxis=+Z  TranslationStandardOffset=0  TranslationStandardOffsetUnits=m  TranslationROffset=0  TranslationROffsetUnits=m  TranslationThetaOffset=0  TranslationThetaOffsetUnits=deg  TranslationZOffset=0  TranslationZOffsetUnits=m
  Transform Camera RR : sm_lib/Frames and Transforms/Rigid Transform  RotationMethod=StandardAxis  FollAlignAxisA=+X  BaseAlignAxisA=+Y  FollAlignAxisB=+Y  BaseAlignAxisB=+Z  RotationStandardAxis=+Z  RotationAngle=+15+90  RotationAngleUnits=deg  RotationArbitraryAxis=[0 0 1]  RotationSequenceAxes=FollowerAxes  RotationSequence=XYX  RotationSequenceAngles=[0 0 0]  RotationSequenceAnglesUnits=deg  RotationMatrix=[1 0 0; 0 1 0; 0 0 1]  Quaternion=[1 0 0 0]  TranslationMethod=Cartesian  TranslationCartesianOffset=[1.5 -4 0.75]  TranslationCartesianOffsetUnits=m  TranslationStandardAxis=+Z  TranslationStandardOffset=0  TranslationStandardOffsetUnits=m  TranslationROffset=0  TranslationROffsetUnits=m  TranslationThetaOffset=0  TranslationThetaOffsetUnits=deg  TranslationZOffset=0  TranslationZOffsetUnits=m
  Transform Camera Rear : sm_lib/Frames and Transforms/Rigid Transform  RotationMethod=None  FollAlignAxisA=+X  BaseAlignAxisA=+Y  FollAlignAxisB=+Y  BaseAlignAxisB=+Z  RotationStandardAxis=+Z  RotationAngle=0.0  RotationAngleUnits=deg  RotationArbitraryAxis=[0 0 1]  RotationSequenceAxes=FollowerAxes  RotationSequence=XYX  RotationSequenceAngles=[0 0 0]  RotationSequenceAnglesUnits=deg  RotationMatrix=[1 0 0; 0 1 0; 0 0 1]  Quaternion=[1 0 0 0]  TranslationMethod=Cartesian  TranslationCartesianOffset=[0 -4.75 1.00]  TranslationCartesianOffsetUnits=m  TranslationStandardAxis=+Z  TranslationStandardOffset=0  TranslationStandardOffsetUnits=m  TranslationROffset=0  TranslationROffsetUnits=m  TranslationThetaOffset=0  TranslationThetaOffsetUnits=deg  TranslationZOffset=0  TranslationZOffsetUnits=m
  Transform Camera Right : sm_lib/Frames and Transforms/Rigid Transform  RotationMethod=None  FollAlignAxisA=+X  BaseAlignAxisA=+Y  FollAlignAxisB=+Y  BaseAlignAxisB=+Z  RotationStandardAxis=+Z  RotationAngle=0.0  RotationAngleUnits=deg  RotationArbitraryAxis=[0 0 1]  RotationSequenceAxes=FollowerAxes  RotationSequence=XYX  RotationSequenceAngles=[0 0 0]  RotationSequenceAnglesUnits=deg  RotationMatrix=[1 0 0; 0 1 0; 0 0 1]  Quaternion=[1 0 0 0]  TranslationMethod=Cartesian  TranslationCartesianOffset=[4 0.45 0.5]  TranslationCartesianOffsetUnits=m  TranslationStandardAxis=+Z  TranslationStandardOffset=0  TranslationStandardOffsetUnits=m  TranslationROffset=0  TranslationROffsetUnits=m  TranslationThetaOffset=0  TranslationThetaOffsetUnits=deg  TranslationZOffset=0  TranslationZOffsetUnits=m
  Transform Camera Roof : sm_lib/Frames and Transforms/Rigid Transform  RotationMethod=StandardAxis  FollAlignAxisA=+X  BaseAlignAxisA=+Y  FollAlignAxisB=+Y  BaseAlignAxisB=+Z  RotationStandardAxis=+X  RotationAngle=-20  RotationAngleUnits=deg  RotationArbitraryAxis=[0 0 1]  RotationSequenceAxes=FollowerAxes  RotationSequence=XYX  RotationSequenceAngles=[0 0 0]  RotationSequenceAnglesUnits=deg  RotationMatrix=[1 0 0; 0 1 0; 0 0 1]  Quaternion=[1 0 0 0]  TranslationMethod=Cartesian  TranslationCartesianOffset=[0 -0.35 2]  TranslationCartesianOffsetUnits=m  TranslationStandardAxis=+Z  TranslationStandardOffset=0  TranslationStandardOffsetUnits=m  TranslationROffset=0  TranslationROffsetUnits=m  TranslationThetaOffset=0  TranslationThetaOffsetUnits=deg  TranslationZOffset=0  TranslationZOffsetUnits=m
  Transform Camera WhlFR : sm_lib/Frames and Transforms/Rigid Transform  RotationMethod=RotationSequence  FollAlignAxisA=+X  BaseAlignAxisA=+Y  FollAlignAxisB=+Y  BaseAlignAxisB=+Z  RotationStandardAxis=+Z  RotationAngle=0.0  RotationAngleUnits=deg  RotationArbitraryAxis=[0 0 1]  RotationSequenceAxes=FollowerAxes  RotationSequence=ZYX  RotationSequenceAngles=[45 0 0]  RotationSequenceAnglesUnits=deg  RotationMatrix=[1 0 0; 0 1 0; 0 0 1]  Quaternion=[1 0 0 0]  TranslationMethod=Cartesian  TranslationCartesianOffset=[1.6 2.0 -0.15]  TranslationCartesianOffsetUnits=m  TranslationStandardAxis=+Z  TranslationStandardOffset=0  TranslationStandardOffsetUnits=m  TranslationROffset=0  TranslationROffsetUnits=m  TranslationThetaOffset=0  TranslationThetaOffsetUnits=deg  TranslationZOffset=0  TranslationZOffsetUnits=m
  H : PMIOPort  Side=Left
  connections:
  Reference Camera Roof/RConn1 -- Transform Camera Roof/RConn1
  Reference Camera ImplRR/RConn1 -- Transform Camera ImplRR/RConn1
  Reference Camera Rear/RConn1 -- Transform Camera Rear/RConn1
  Reference Camera RR/RConn1 -- Transform Camera RR/RConn1
  Reference Camera Cab/RConn1 -- Transform Camera Cab/RConn1
  Transform Camera Cab/LConn1 -- Transform Camera IsoFR/LConn1 -- Transform Camera WhlFR/LConn1 -- Transform Camera LinkageR/LConn1 -- Transform Camera Rear/LConn1 -- Transform Camera Right/LConn1 -- Transform Camera RR/LConn1 -- Transform Camera ImplRR/LConn1 -- Transform Camera Roof/LConn1 -- H/RConn1
  Transform Camera Right/RConn1 -- Reference Camera Right/RConn1
  Reference Camera LinkageR/RConn1 -- Transform Camera LinkageR/RConn1
  Reference Camera WhlFR/RConn1 -- Transform Camera WhlFR/RConn1
  Reference Camera IsoFR/RConn1 -- Transform Camera IsoFR/RConn1

== system sm_wheel_loader_lib/Wheel Loader Vehicle/Frame Front/Fender FL ==
  Fender FL : sm_lib/Body Elements/File Solid  ExtGeomFileName=FrameF_FenderFL.STEP  UnitType=FromFile  ExtGeomFileUnits=m  StepReaderType=HEX  ExportConvexHullGeometry=off  InertiaType=Custom  BasedOnType=DensityFromFile  Density=1000  DensityUnits=kg/m^3  Mass=Wheel_Loader.bodyGroups(29).subGroups(1).inertialProperties.mass  MassUnits=kg  CenterOfMass=Wheel_Loader.bodyGroups(29).subGroups(1).inertialProperties.centerOfMass  CenterOfMassUnits=m  MomentsOfInertia=Wheel_Loader.bodyGroups(29).subGroups(1).inertialProperties.momentsOfInertia  MomentsOfInertiaUnits=kg*m^2  ProductsOfInertia=Wheel_Loader.bodyGroups(29).subGroups(1).inertialProperties.productsOfInertia  ProductsOfInertiaUnits=kg*m^2  GraphicType=FromGeometry  MarkerShape=Sphere  MarkerSize=10  GraphicVisPropType=SimpleVisualProperties  GraphicDiffuseColor=Wheel_Loader.bodyGroups(29).subGroups(1).visualProperties.rgb  GraphicOpacity=Wheel_Loader.bodyGroups(29).subGroups(1).visualProperties.opacity  GraphicSpecularColor=[0.5 0.5 0.5 1.0]  GraphicAmbientColor=[0.15 0.15 0.15 1.0]  GraphicEmissiveColor=[0.0 0.0 0.0 1.0]  GraphicShininess=75  DoExposeReferenceFrame=on  SerializedFrames=<Frames/>
  RT_FrontFrame_LFFender_Weld : sm_lib/Frames and Transforms/Rigid Transform  RotationMethod=RotationMatrix  FollAlignAxisA=+X  BaseAlignAxisA=+Y  FollAlignAxisB=+Y  BaseAlignAxisB=+Z  RotationStandardAxis=+Z  RotationAngle=0.0  RotationAngleUnits=deg  RotationArbitraryAxis=[0 0 1]  RotationSequenceAxes=FollowerAxes  RotationSequence=XYX  RotationSequenceAngles=[0 0 0]  RotationSequenceAnglesUnits=deg  RotationMatrix=[1 0 0; 0 1 0; 0 0 1]  Quaternion=[1 0 0 0]  TranslationMethod=Cartesian  TranslationCartesianOffset=[0 0 0]  TranslationCartesianOffsetUnits=m  TranslationStandardAxis=+Z  TranslationStandardOffset=0  TranslationStandardOffsetUnits=m  TranslationROffset=0  TranslationROffsetUnits=m  TranslationThetaOffset=0  TranslationThetaOffsetUnits=deg  TranslationZOffset=0  TranslationZOffsetUnits=m
  B1 : PMIOPort  Side=Left
  connections:
  Fender FL/RConn1 -- RT_FrontFrame_LFFender_Weld/LConn1
  RT_FrontFrame_LFFender_Weld/RConn1 -- B1/RConn1

== system sm_wheel_loader_lib/Wheel Loader Vehicle/Frame Front/Fender FR ==
  Fender FR : sm_lib/Body Elements/File Solid  ExtGeomFileName=FrameF_FenderFR.STEP  UnitType=FromFile  ExtGeomFileUnits=m  StepReaderType=HEX  ExportConvexHullGeometry=off  InertiaType=Custom  BasedOnType=DensityFromFile  Density=1000  DensityUnits=kg/m^3  Mass=Wheel_Loader.bodyGroups(28).subGroups(1).inertialProperties.mass  MassUnits=kg  CenterOfMass=Wheel_Loader.bodyGroups(28).subGroups(1).inertialProperties.centerOfMass  CenterOfMassUnits=m  MomentsOfInertia=Wheel_Loader.bodyGroups(28).subGroups(1).inertialProperties.momentsOfInertia  MomentsOfInertiaUnits=kg*m^2  ProductsOfInertia=Wheel_Loader.bodyGroups(28).subGroups(1).inertialProperties.productsOfInertia  ProductsOfInertiaUnits=kg*m^2  GraphicType=FromGeometry  MarkerShape=Sphere  MarkerSize=10  GraphicVisPropType=SimpleVisualProperties  GraphicDiffuseColor=Wheel_Loader.bodyGroups(28).subGroups(1).visualProperties.rgb  GraphicOpacity=Wheel_Loader.bodyGroups(28).subGroups(1).visualProperties.opacity  GraphicSpecularColor=[0.5 0.5 0.5 1.0]  GraphicAmbientColor=[0.15 0.15 0.15 1.0]  GraphicEmissiveColor=[0.0 0.0 0.0 1.0]  GraphicShininess=75  DoExposeReferenceFrame=on  SerializedFrames=<Frames/>
  RT_FrontFrame_RFFender_Weld : sm_lib/Frames and Transforms/Rigid Transform  RotationMethod=RotationMatrix  FollAlignAxisA=+X  BaseAlignAxisA=+Y  FollAlignAxisB=+Y  BaseAlignAxisB=+Z  RotationStandardAxis=+Z  RotationAngle=0.0  RotationAngleUnits=deg  RotationArbitraryAxis=[0 0 1]  RotationSequenceAxes=FollowerAxes  RotationSequence=XYX  RotationSequenceAngles=[0 0 0]  RotationSequenceAnglesUnits=deg  RotationMatrix=[1 0 0; 0 1 0; 0 0 1]  Quaternion=[1 0 0 0]  TranslationMethod=Cartesian  TranslationCartesianOffset=[0 0 0]  TranslationCartesianOffsetUnits=m  TranslationStandardAxis=+Z  TranslationStandardOffset=0  TranslationStandardOffsetUnits=m  TranslationROffset=0  TranslationROffsetUnits=m  TranslationThetaOffset=0  TranslationThetaOffsetUnits=deg  TranslationZOffset=0  TranslationZOffsetUnits=m
  B1 : PMIOPort  Side=Left
  connections:
  Fender FR/RConn1 -- RT_FrontFrame_RFFender_Weld/LConn1
  RT_FrontFrame_RFFender_Weld/RConn1 -- B1/RConn1
